simulink model "pid_adrc_duibi"  (R2023b)
settings: Solver=VariableStepAuto  StartTime=0.0  StopTime=10.0  RelTol=1e-3
values from neighbouring files (symbols this model uses):
  gama = 0.003    [startup.m]
  ke = 78.4    [startup.m]
  kf = 96.0    (= 96)    [startup.m]
  kii = 1061*R    (= 19755.82)    [startup.m]
  kiv = kpv*100    (= 7015.3125)    [startup.m]
  kp = 150    [startup.m]
  kpi = 1061*L    (= 16265.13)    [startup.m]
  kpv = 100*6*J/(kf)    (= 70.153125)    [startup.m]
  L = 15.33    [startup.m]
  R = 18.62    [startup.m]
  r = 10    [startup.m]
  tao = 0.003    [startup.m]
  U = m2^2*y^2+2*m1*m2*y^2+I1*(m1+m2)    [startup.m]
undefined symbols (not defined in the file or in its folder): sigbuilder_block
libraries: slpidlib x42, simulink x18
(part 2 of 2)

== system pid_adrc_duibi/Signal Builder1 ==
  Demux : Demux  Tag=STV Demux  Outputs=1
      settings: DisplayOption=none
  FromWs : FromWorkspace  Tag=STV FromWs  VariableName=tuvar
      SigBuilderData=|
      | common.afterFinalStr = 'Extrapolate'
      | common.sampleTime = 0
      | dataSet.timeRange = [0 10]
      | dataSet.name = 'Group 1'
      | sbobj.Groups.Name = 'Group 1'
      | sbobj.Groups.Signals.Name = 'Signal 1'
      | sbobj.Groups.Signals.XData = [0 1 2 8 9 10]
      | sbobj.Groups.Signals.YData = [0 0 1 1 1 1]
  Signal 1 : Outport  Tag=STV Outport  VectorParamsAs1DForOutWhenUnconnected=off
  wires:
  Demux/1 -> Signal 1/1
  FromWs/1 -> Demux/1

== system pid_adrc_duibi/Signal Builder2 ==
  Demux : Demux  Tag=STV Demux  Outputs=1
      settings: DisplayOption=none
  FromWs : FromWorkspace  Tag=STV FromWs  VariableName=tuvar
      SigBuilderData=|
      | common.afterFinalStr = 'Extrapolate'
      | common.sampleTime = 0
      | dataSet.timeRange = [0 10]
      | dataSet.name = 'Group 1'
      | sbobj.Groups.Name = 'Group 1'
      | sbobj.Groups.Signals.Name = 'Signal 1'
      | sbobj.Groups.Signals.XData = [0 1 2 8 9 10]
      | sbobj.Groups.Signals.YData = [0 0 1 1 1 1]
  Signal 1 : Outport  Tag=STV Outport  VectorParamsAs1DForOutWhenUnconnected=off
  wires:
  Demux/1 -> Signal 1/1
  FromWs/1 -> Demux/1

== system pid_adrc_duibi/Signal Builder3 ==
  Demux : Demux  Tag=STV Demux  Outputs=1
      settings: DisplayOption=none
  FromWs : FromWorkspace  Tag=STV FromWs  VariableName=tuvar
      SigBuilderData=|
      | common.afterFinalStr = 'Extrapolate'
      | common.sampleTime = 0
      | dataSet.timeRange = [0 10]
      | dataSet.name = 'Group 1'
      | sbobj.Groups.Name = 'Group 1'
      | sbobj.Groups.Signals.Name = 'Signal 1'
      | sbobj.Groups.Signals.XData = [0 1 2 8 9 10]
      | sbobj.Groups.Signals.YData = [0 0 1 1 1 1]
  Signal 1 : Outport  Tag=STV Outport  VectorParamsAs1DForOutWhenUnconnected=off
  wires:
  Demux/1 -> Signal 1/1
  FromWs/1 -> Demux/1

== system pid_adrc_duibi/Signal Builder4 ==
  Demux : Demux  Tag=STV Demux  Outputs=1
      settings: DisplayOption=none
  FromWs : FromWorkspace  Tag=STV FromWs  VariableName=tuvar
      SigBuilderData=|
      | common.afterFinalStr = 'Extrapolate'
      | common.sampleTime = 0
      | dataSet.timeRange = [0 10]
      | dataSet.name = 'Group 1'
      | sbobj.Groups.Name = 'Group 1'
      | sbobj.Groups.Signals.Name = 'Signal 1'
      | sbobj.Groups.Signals.XData = [0 1 2 8 9 10]
      | sbobj.Groups.Signals.YData = [0 0 1 1 1 1]
  Signal 1 : Outport  Tag=STV Outport  VectorParamsAs1DForOutWhenUnconnected=off
  wires:
  Demux/1 -> Signal 1/1
  FromWs/1 -> Demux/1

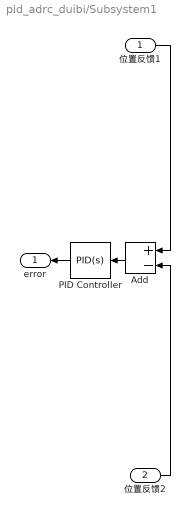
== system pid_adrc_duibi/Subsystem1 ==
  位置反馈1 : Inport
  位置反馈2 : Inport  Port=2
  Add : Sum  Inputs=+-
  PID Controller : simulink/Continuous/PID Controller  Controller=PID  TimeDomain=Continuous-time  SampleTime=-1  IntegratorMethod=Forward Euler  FilterMethod=Forward Euler  Form=Parallel  UseFilter=on  ControllerParametersSource=internal  P=e_kp  I=e_ki  D=e_kd  N=100  InitialConditionSource=internal  InitialConditionForIntegrator=0  InitialConditionForFilter=0  ExternalReset=none  LimitOutput=off  UpperSaturationLimit=inf  LowerSaturationLimit=-inf  LinearizeAsGain=on  AntiWindupMode=none  Kb=1  TrackingMode=off  Kt=1  PParamMin=[]  PParamMax=[]  IParamMin=[]  IParamMax=[]  DParamMin=[]  DParamMax=[]  NParamMin=[]  NParamMax=[]  KbParamMin=[]  KbParamMax=[]  KtParamMin=[]  KtParamMax=[]  POutMin=[]  POutMax=[]  IOutMin=[]  IOutMax=[]  DOutMin=[]  DOutMax=[]  NOutMin=[]  NOutMax=[]  KbOutMin=[]  KbOutMax=[]  KtOutMin=[]  KtOutMax=[]  IntegratorOutMin=[]  IntegratorOutMax=[]  FilterOutMin=[]  FilterOutMax=[]  SumOutMin=[]  SumOutMax=[]  SumI1OutMin=[]  SumI1OutMax=[]  SumI2OutMin=[]  SumI2OutMax=[]  SumI3OutMin=[]  SumI3OutMax=[]  SumDOutMin=[]  SumDOutMax=[]  SaturationOutMin=[]  SaturationOutMax=[]  IntegratorContinuousStateAttributes=''  IntegratorStateMustResolveToSignalObject=off  IntegratorRTWStateStorageClass=Auto  FilterContinuousStateAttributes=''  FilterStateMustResolveToSignalObject=off  FilterRTWStateStorageClass=Auto  DifferentiatorICPrevScaledInput=0  DifferentiatorOutMin=[]  DifferentiatorOutMax=[]  FilterDiffOutCoefMin=[]  FilterDiffOutCoefMax=[]  SumDenOutMin=[]  SumDenOutMax=[]  SumNumOutMin=[]  SumNumOutMax=[]  ReciprocalOutMin=[]  ReciprocalOutMax=[]  DivideOutMin=[]  DivideOutMax=[]  TunerSelectOption=Transfer Function Based (PID Tuner App)
  error : Outport  VectorParamsAs1DForOutWhenUnconnected=off
  wires:
  位置反馈2/1 -> Add/2
  Add/1 -> PID Controller/1
  PID Controller/1 -> error/1
  位置反馈1/1 -> Add/1

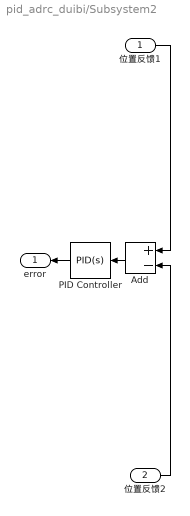
== system pid_adrc_duibi/Subsystem2 ==
  位置反馈1 : Inport
  位置反馈2 : Inport  Port=2
  Add : Sum  Inputs=+-
  PID Controller : slpidlib/PID Controller  Controller=PID  Form=Parallel  TimeDomain=Continuous-time  UseExternalTs=off  SampleTime=-1  IntegratorMethod=Forward Euler  FilterMethod=Forward Euler  ControllerParametersSource=internal  P=e_kp  I=e_ki  UseKiTs=off  D=e_kd  N=100  UseFilter=on  TunerSelectOption=Transfer Function Based (PID Tuner App)  InitialConditionSource=internal  InitialConditionForIntegrator=0  InitialConditionForFilter=0  DifferentiatorICPrevScaledInput=0  ExternalReset=none  TrackingMode=off  Kt=1  LimitOutput=off  SatLimitsSource=internal  UpperSaturationLimit=inf  LowerSaturationLimit=-inf  LinearizeAsGain=on  AntiWindupMode=none  Kb=1  LimitIntegrator=off  UpperIntegratorSaturationLimit=inf  LowerIntegratorSaturationLimit=-inf  POutMin=[]  POutMax=[]  IOutMin=[]  IOutMax=[]  DOutMin=[]  DOutMax=[]  NOutMin=[]  NOutMax=[]  SumOutMin=[]  SumOutMax=[]  SaturationOutMin=[]  SaturationOutMax=[]  PParamMin=[]  PParamMax=[]  IParamMin=[]  IParamMax=[]  DParamMin=[]  DParamMax=[]  NParamMin=[]  NParamMax=[]  KbParamMin=[]  KbParamMax=[]  KtParamMin=[]  KtParamMax=[]  KbOutMin=[]  KbOutMax=[]  KtOutMin=[]  KtOutMax=[]  IntegratorOutMin=[]  IntegratorOutMax=[]  FilterOutMin=[]  FilterOutMax=[]  SumI1OutMin=[]  SumI1OutMax=[]  SumI2OutMin=[]  SumI2OutMax=[]  SumI3OutMin=[]  SumI3OutMax=[]  SumI4OutMin=[]  SumI4OutMax=[]  SumDOutMin=[]  SumDOutMax=[]  DifferentiatorOutMin=[]  DifferentiatorOutMax=[]  FilterDiffOutCoefMin=[]  FilterDiffOutCoefMax=[]  ReciprocalOutMin=[]  ReciprocalOutMax=[]  SumDenOutMin=[]  SumDenOutMax=[]  SumNumOutMin=[]  SumNumOutMax=[]  DivideOutMin=[]  DivideOutMax=[]  UdiffTsProdOutMin=[]  UdiffTsProdOutMax=[]  NTsProdOutMin=[]  NTsProdOutMax=[]  UintegralTsProdOutMin=[]  UintegralTsProdOutMax=[]  UngainTsProdOutMin=[]  UngainTsProdOutMax=[]  ClampingZeroOutDataTypeStr=Inherit: Inherit via back propagation  ClampingZeroOutMin=[]  ClampingZeroOutMax=[]  FilterDenConstantOutDataTypeStr=Inherit: Inherit via back propagation  FilterDenConstantOutMin=[]  FilterDenConstantOutMax=[]  PCopyOutDataTypeStr=Inherit: Inherit via back propagation  PCopyOutMin=[]  PCopyOutMax=[]  NCopyOutDataTypeStr=Inherit: Inherit via back propagation  NCopyOutMin=[]  NCopyOutMax=[]  IntegratorContinuousStateAttributes=''  IntegratorStateMustResolveToSignalObject=off  IntegratorRTWStateStorageClass=Auto  FilterContinuousStateAttributes=''  FilterStateMustResolveToSignalObject=off  FilterRTWStateStorageClass=Auto  ParallelPVariant=InternalParameters  IdealPVariant=Disabled  IVariant=InternalParameters  DVariant=InternalParameters  IntegratorVariant=Continuous  SatVariant=Disabled  AWVariant=Passthrough  PCopyVariant=Disabled  TRVariant=Disabled  FdbkBlocksVariant=Forward  IdealPFdbkVariant=Disabled  SatFdbkVariant=Disabled  DerivativeFilterVariant=ContFilter  NVariant=InternalParameters  NCopyVariant=Disabled  FilterICVariant=InternalICsFilter  IntegratorICVariant=InternalICs  ExternalResetVariant=Disabled  TRSumVariant=Passthrough  SumFdbkVariant=Disabled  SumVariant=Sum_PID  TsampFilterVariant=InternalTs  TsampNgainVariant=Passthrough  TsampIntegralVariant=Disabled_SignalSpec  ExternalSaturationOutDataTypeStr=Inherit: Same as second input
  error : Outport  VectorParamsAs1DForOutWhenUnconnected=off
  wires:
  位置反馈2/1 -> Add/2
  Add/1 -> PID Controller/1
  PID Controller/1 -> error/1
  位置反馈1/1 -> Add/1

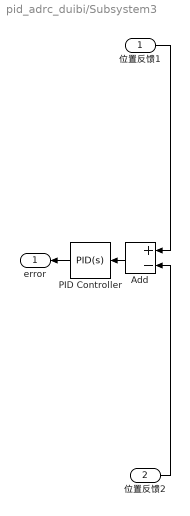
== system pid_adrc_duibi/Subsystem3 ==
  位置反馈1 : Inport
  位置反馈2 : Inport  Port=2
  Add : Sum  Inputs=+-
  PID Controller : slpidlib/PID Controller  Controller=PID  Form=Parallel  TimeDomain=Continuous-time  UseExternalTs=off  SampleTime=-1  IntegratorMethod=Forward Euler  FilterMethod=Forward Euler  ControllerParametersSource=internal  P=e_kp  I=e_ki  UseKiTs=off  D=e_kd  N=100  UseFilter=on  TunerSelectOption=Transfer Function Based (PID Tuner App)  InitialConditionSource=internal  InitialConditionForIntegrator=0  InitialConditionForFilter=0  DifferentiatorICPrevScaledInput=0  ExternalReset=none  TrackingMode=off  Kt=1  LimitOutput=off  SatLimitsSource=internal  UpperSaturationLimit=inf  LowerSaturationLimit=-inf  LinearizeAsGain=on  AntiWindupMode=none  Kb=1  LimitIntegrator=off  UpperIntegratorSaturationLimit=inf  LowerIntegratorSaturationLimit=-inf  POutMin=[]  POutMax=[]  IOutMin=[]  IOutMax=[]  DOutMin=[]  DOutMax=[]  NOutMin=[]  NOutMax=[]  SumOutMin=[]  SumOutMax=[]  SaturationOutMin=[]  SaturationOutMax=[]  PParamMin=[]  PParamMax=[]  IParamMin=[]  IParamMax=[]  DParamMin=[]  DParamMax=[]  NParamMin=[]  NParamMax=[]  KbParamMin=[]  KbParamMax=[]  KtParamMin=[]  KtParamMax=[]  KbOutMin=[]  KbOutMax=[]  KtOutMin=[]  KtOutMax=[]  IntegratorOutMin=[]  IntegratorOutMax=[]  FilterOutMin=[]  FilterOutMax=[]  SumI1OutMin=[]  SumI1OutMax=[]  SumI2OutMin=[]  SumI2OutMax=[]  SumI3OutMin=[]  SumI3OutMax=[]  SumI4OutMin=[]  SumI4OutMax=[]  SumDOutMin=[]  SumDOutMax=[]  DifferentiatorOutMin=[]  DifferentiatorOutMax=[]  FilterDiffOutCoefMin=[]  FilterDiffOutCoefMax=[]  ReciprocalOutMin=[]  ReciprocalOutMax=[]  SumDenOutMin=[]  SumDenOutMax=[]  SumNumOutMin=[]  SumNumOutMax=[]  DivideOutMin=[]  DivideOutMax=[]  UdiffTsProdOutMin=[]  UdiffTsProdOutMax=[]  NTsProdOutMin=[]  NTsProdOutMax=[]  UintegralTsProdOutMin=[]  UintegralTsProdOutMax=[]  UngainTsProdOutMin=[]  UngainTsProdOutMax=[]  ClampingZeroOutDataTypeStr=Inherit: Inherit via back propagation  ClampingZeroOutMin=[]  ClampingZeroOutMax=[]  FilterDenConstantOutDataTypeStr=Inherit: Inherit via back propagation  FilterDenConstantOutMin=[]  FilterDenConstantOutMax=[]  PCopyOutDataTypeStr=Inherit: Inherit via back propagation  PCopyOutMin=[]  PCopyOutMax=[]  NCopyOutDataTypeStr=Inherit: Inherit via back propagation  NCopyOutMin=[]  NCopyOutMax=[]  IntegratorContinuousStateAttributes=''  IntegratorStateMustResolveToSignalObject=off  IntegratorRTWStateStorageClass=Auto  FilterContinuousStateAttributes=''  FilterStateMustResolveToSignalObject=off  FilterRTWStateStorageClass=Auto  ParallelPVariant=InternalParameters  IdealPVariant=Disabled  IVariant=InternalParameters  DVariant=InternalParameters  IntegratorVariant=Continuous  SatVariant=Disabled  AWVariant=Passthrough  PCopyVariant=Disabled  TRVariant=Disabled  FdbkBlocksVariant=Forward  IdealPFdbkVariant=Disabled  SatFdbkVariant=Disabled  DerivativeFilterVariant=ContFilter  NVariant=InternalParameters  NCopyVariant=Disabled  FilterICVariant=InternalICsFilter  IntegratorICVariant=InternalICs  ExternalResetVariant=Disabled  TRSumVariant=Passthrough  SumFdbkVariant=Disabled  SumVariant=Sum_PID  TsampFilterVariant=InternalTs  TsampNgainVariant=Passthrough  TsampIntegralVariant=Disabled_SignalSpec  ExternalSaturationOutDataTypeStr=Inherit: Same as second input
  error : Outport  VectorParamsAs1DForOutWhenUnconnected=off
  wires:
  位置反馈2/1 -> Add/2
  Add/1 -> PID Controller/1
  PID Controller/1 -> error/1
  位置反馈1/1 -> Add/1

== system pid_adrc_duibi/Subsystem4 ==
  位置反馈1 : Inport
  位置反馈2 : Inport  Port=2
  Add : Sum  Inputs=+-
  PID Controller : simulink/Continuous/PID Controller  Controller=PID  TimeDomain=Continuous-time  SampleTime=-1  IntegratorMethod=Forward Euler  FilterMethod=Forward Euler  Form=Parallel  UseFilter=on  ControllerParametersSource=internal  P=e_kp  I=e_ki  D=e_kd  N=100  InitialConditionSource=internal  InitialConditionForIntegrator=0  InitialConditionForFilter=0  ExternalReset=none  LimitOutput=off  UpperSaturationLimit=inf  LowerSaturationLimit=-inf  LinearizeAsGain=on  AntiWindupMode=none  Kb=1  TrackingMode=off  Kt=1  PParamMin=[]  PParamMax=[]  IParamMin=[]  IParamMax=[]  DParamMin=[]  DParamMax=[]  NParamMin=[]  NParamMax=[]  KbParamMin=[]  KbParamMax=[]  KtParamMin=[]  KtParamMax=[]  POutMin=[]  POutMax=[]  IOutMin=[]  IOutMax=[]  DOutMin=[]  DOutMax=[]  NOutMin=[]  NOutMax=[]  KbOutMin=[]  KbOutMax=[]  KtOutMin=[]  KtOutMax=[]  IntegratorOutMin=[]  IntegratorOutMax=[]  FilterOutMin=[]  FilterOutMax=[]  SumOutMin=[]  SumOutMax=[]  SumI1OutMin=[]  SumI1OutMax=[]  SumI2OutMin=[]  SumI2OutMax=[]  SumI3OutMin=[]  SumI3OutMax=[]  SumDOutMin=[]  SumDOutMax=[]  SaturationOutMin=[]  SaturationOutMax=[]  IntegratorContinuousStateAttributes=''  IntegratorStateMustResolveToSignalObject=off  IntegratorRTWStateStorageClass=Auto  FilterContinuousStateAttributes=''  FilterStateMustResolveToSignalObject=off  FilterRTWStateStorageClass=Auto  DifferentiatorICPrevScaledInput=0  DifferentiatorOutMin=[]  DifferentiatorOutMax=[]  FilterDiffOutCoefMin=[]  FilterDiffOutCoefMax=[]  SumDenOutMin=[]  SumDenOutMax=[]  SumNumOutMin=[]  SumNumOutMax=[]  ReciprocalOutMin=[]  ReciprocalOutMax=[]  DivideOutMin=[]  DivideOutMax=[]  TunerSelectOption=Transfer Function Based (PID Tuner App)
  error : Outport  VectorParamsAs1DForOutWhenUnconnected=off
  wires:
  位置反馈2/1 -> Add/2
  Add/1 -> PID Controller/1
  PID Controller/1 -> error/1
  位置反馈1/1 -> Add/1

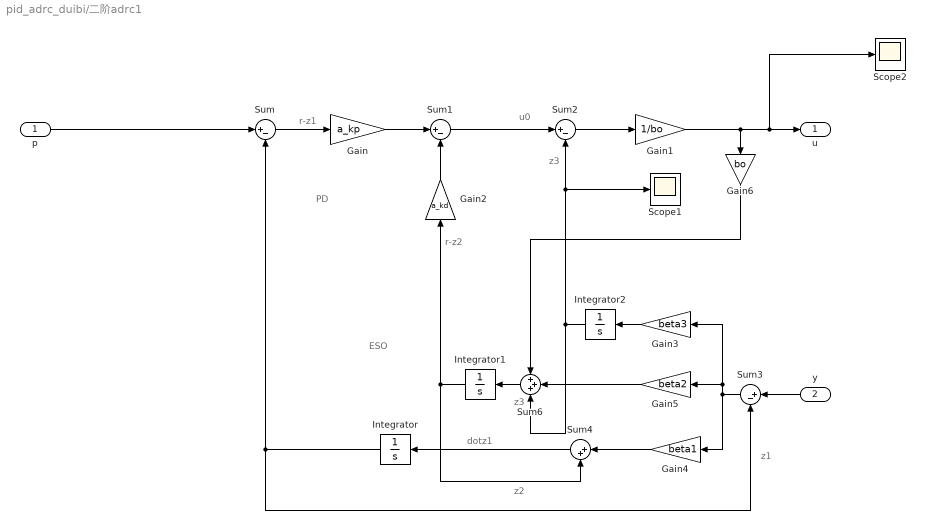
== system pid_adrc_duibi/二阶adrc1 ==
  note: ESO
  note: PD
  note: z3
  note: dotz1
  note: z2
  note: z1
  note: z3
  note: u0
  note: r-z2
  note: r-z1
  p : Inport
  y : Inport  Port=2
  Gain : Gain  Gain=a_kp
  Gain1 : Gain  Gain=1/bo
  Gain2 : Gain  Gain=a_kd
  Gain3 : Gain  Gain=beta3
  Gain4 : Gain  Gain=beta1
  Gain5 : Gain  Gain=beta2
  Gain6 : Gain  Gain=bo
  Integrator : Integrator
  Integrator1 : Integrator
  Integrator2 : Integrator
  Scope1 : Scope
  Scope2 : Scope
  Sum{,1..3} (4 alike) : Sum  Inputs=|+-
  Sum4 : Sum  Inputs=|++
  Sum6 : Sum  Inputs=+++
  u : Outport  VectorParamsAs1DForOutWhenUnconnected=off
  wires:
  p/1 -> Sum/1
  Sum/1 -> Gain/1
  Gain/1 -> Sum1/1
  Gain2/1 -> Sum1/2
  Sum2/1 -> Gain1/1
  Gain1/1 -> Gain6/1, Scope2/1, u/1
  Integrator/1 -> Sum/2, Sum3/2
  y/1 -> Sum3/1
  Sum3/1 -> Gain4/1, Gain3/1, Gain5/1
  Gain4/1 -> Sum4/1
  Sum4/1 -> Integrator/1
  Gain5/1 -> Sum6/2
  Gain6/1 -> Sum6/1
  Integrator2/1 -> Sum6/3, Sum2/2, Scope1/1
  Sum6/1 -> Integrator1/1
  Gain3/1 -> Integrator2/1
  Integrator1/1 -> Gain2/1, Sum4/2
  Sum1/1 -> Sum2/1

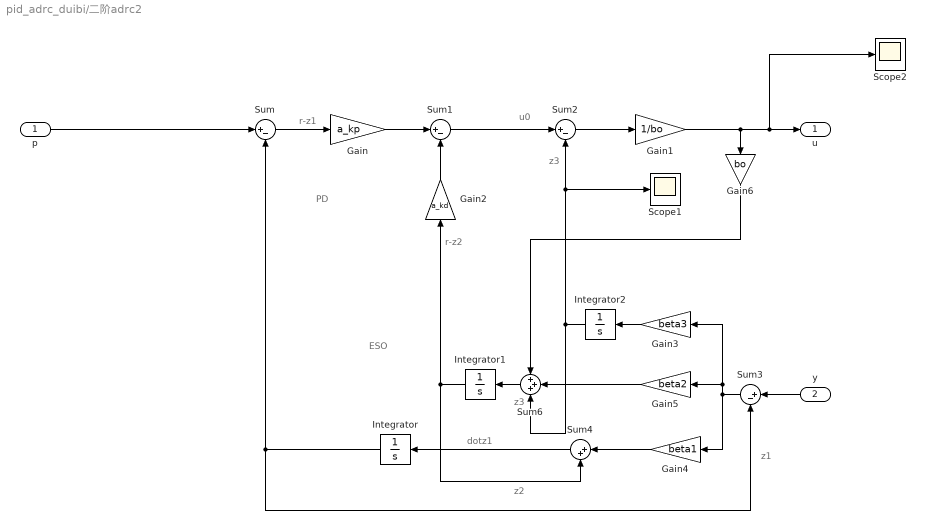
== system pid_adrc_duibi/二阶adrc2 ==
  note: ESO
  note: PD
  note: z3
  note: dotz1
  note: z2
  note: z1
  note: z3
  note: u0
  note: r-z2
  note: r-z1
  p : Inport
  y : Inport  Port=2
  Gain : Gain  Gain=a_kp
  Gain1 : Gain  Gain=1/bo
  Gain2 : Gain  Gain=a_kd
  Gain3 : Gain  Gain=beta3
  Gain4 : Gain  Gain=beta1
  Gain5 : Gain  Gain=beta2
  Gain6 : Gain  Gain=bo
  Integrator : Integrator
  Integrator1 : Integrator
  Integrator2 : Integrator
  Scope1 : Scope
  Scope2 : Scope
  Sum{,1..3} (4 alike) : Sum  Inputs=|+-
  Sum4 : Sum  Inputs=|++
  Sum6 : Sum  Inputs=+++
  u : Outport  VectorParamsAs1DForOutWhenUnconnected=off
  wires:
  p/1 -> Sum/1
  Sum/1 -> Gain/1
  Gain/1 -> Sum1/1
  Gain2/1 -> Sum1/2
  Sum2/1 -> Gain1/1
  Gain1/1 -> Gain6/1, Scope2/1, u/1
  Integrator/1 -> Sum/2, Sum3/2
  y/1 -> Sum3/1
  Sum3/1 -> Gain4/1, Gain3/1, Gain5/1
  Gain4/1 -> Sum4/1
  Sum4/1 -> Integrator/1
  Gain5/1 -> Sum6/2
  Gain6/1 -> Sum6/1
  Integrator2/1 -> Sum6/3, Sum2/2, Scope1/1
  Sum6/1 -> Integrator1/1
  Gain3/1 -> Integrator2/1
  Sum1/1 -> Sum2/1
  Integrator1/1 -> Gain2/1, Sum4/2

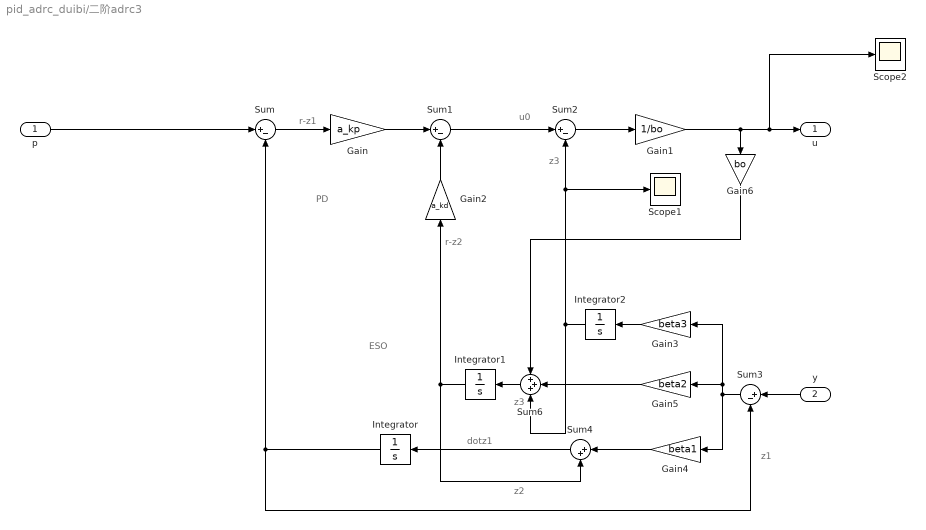
== system pid_adrc_duibi/二阶adrc3 ==
  note: ESO
  note: PD
  note: z3
  note: dotz1
  note: z2
  note: z1
  note: z3
  note: u0
  note: r-z2
  note: r-z1
  p : Inport
  y : Inport  Port=2
  Gain : Gain  Gain=a_kp
  Gain1 : Gain  Gain=1/bo
  Gain2 : Gain  Gain=a_kd
  Gain3 : Gain  Gain=beta3
  Gain4 : Gain  Gain=beta1
  Gain5 : Gain  Gain=beta2
  Gain6 : Gain  Gain=bo
  Integrator : Integrator
  Integrator1 : Integrator
  Integrator2 : Integrator
  Scope1 : Scope
  Scope2 : Scope
  Sum{,1..3} (4 alike) : Sum  Inputs=|+-
  Sum4 : Sum  Inputs=|++
  Sum6 : Sum  Inputs=+++
  u : Outport  VectorParamsAs1DForOutWhenUnconnected=off
  wires:
  p/1 -> Sum/1
  Sum/1 -> Gain/1
  Gain/1 -> Sum1/1
  Gain2/1 -> Sum1/2
  Sum2/1 -> Gain1/1
  Gain1/1 -> Gain6/1, Scope2/1, u/1
  Integrator/1 -> Sum/2, Sum3/2
  y/1 -> Sum3/1
  Sum3/1 -> Gain4/1, Gain3/1, Gain5/1
  Gain4/1 -> Sum4/1
  Sum4/1 -> Integrator/1
  Gain5/1 -> Sum6/2
  Gain6/1 -> Sum6/1
  Integrator2/1 -> Sum6/3, Sum2/2, Scope1/1
  Sum6/1 -> Integrator1/1
  Gain3/1 -> Integrator2/1
  Integrator1/1 -> Gain2/1, Sum4/2
  Sum1/1 -> Sum2/1

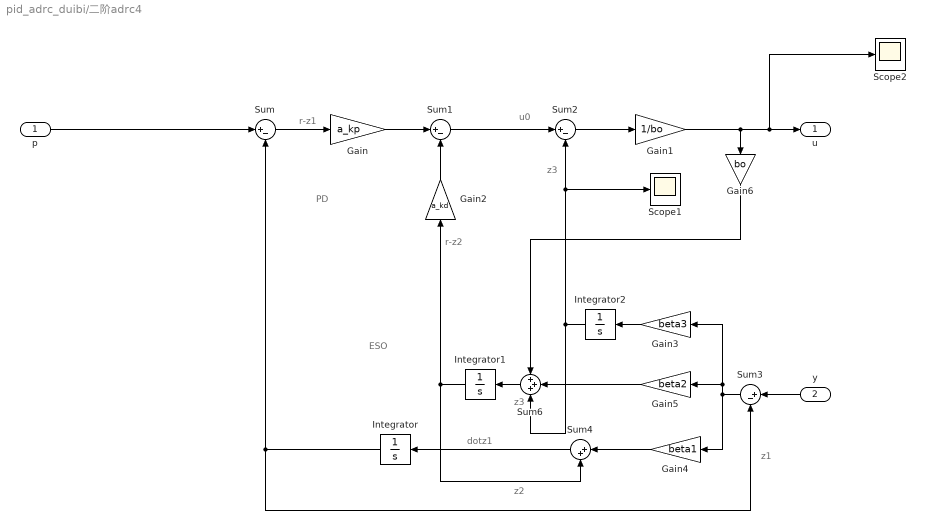
== system pid_adrc_duibi/二阶adrc4 ==
  note: ESO
  note: PD
  note: z3
  note: dotz1
  note: z2
  note: z1
  note: z3
  note: u0
  note: r-z2
  note: r-z1
  p : Inport
  y : Inport  Port=2
  Gain : Gain  Gain=a_kp
  Gain1 : Gain  Gain=1/bo
  Gain2 : Gain  Gain=a_kd
  Gain3 : Gain  Gain=beta3
  Gain4 : Gain  Gain=beta1
  Gain5 : Gain  Gain=beta2
  Gain6 : Gain  Gain=bo
  Integrator : Integrator
  Integrator1 : Integrator
  Integrator2 : Integrator
  Scope1 : Scope
  Scope2 : Scope
  Sum{,1..3} (4 alike) : Sum  Inputs=|+-
  Sum4 : Sum  Inputs=|++
  Sum6 : Sum  Inputs=+++
  u : Outport  VectorParamsAs1DForOutWhenUnconnected=off
  wires:
  Sum/1 -> Gain/1
  Gain/1 -> Sum1/1
  Gain2/1 -> Sum1/2
  Sum2/1 -> Gain1/1
  Gain1/1 -> Gain6/1, Scope2/1, u/1
  Integrator/1 -> Sum/2, Sum3/2
  y/1 -> Sum3/1
  Sum3/1 -> Gain4/1, Gain3/1, Gain5/1
  Gain4/1 -> Sum4/1
  Sum4/1 -> Integrator/1
  Gain5/1 -> Sum6/2
  Gain6/1 -> Sum6/1
  Integrator2/1 -> Sum6/3, Sum2/2, Scope1/1
  Sum6/1 -> Integrator1/1
  Gain3/1 -> Integrator2/1
  Integrator1/1 -> Gain2/1, Sum4/2
  p/1 -> Sum/1
  Sum1/1 -> Sum2/1

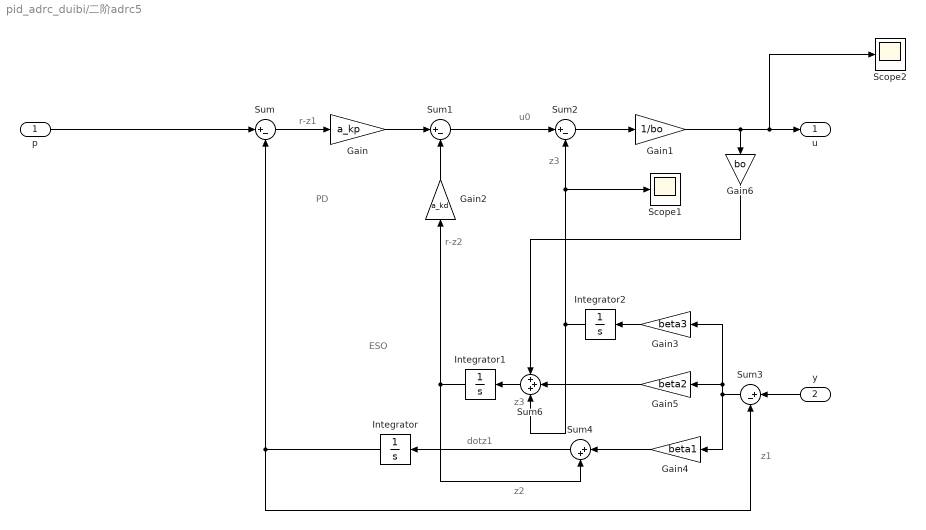
== system pid_adrc_duibi/二阶adrc5 ==
  note: ESO
  note: PD
  note: z3
  note: dotz1
  note: z2
  note: z1
  note: z3
  note: u0
  note: r-z2
  note: r-z1
  p : Inport
  y : Inport  Port=2
  Gain : Gain  Gain=a_kp
  Gain1 : Gain  Gain=1/bo
  Gain2 : Gain  Gain=a_kd
  Gain3 : Gain  Gain=beta3
  Gain4 : Gain  Gain=beta1
  Gain5 : Gain  Gain=beta2
  Gain6 : Gain  Gain=bo
  Integrator : Integrator
  Integrator1 : Integrator
  Integrator2 : Integrator
  Scope1 : Scope
  Scope2 : Scope
  Sum{,1..3} (4 alike) : Sum  Inputs=|+-
  Sum4 : Sum  Inputs=|++
  Sum6 : Sum  Inputs=+++
  u : Outport  VectorParamsAs1DForOutWhenUnconnected=off
  wires:
  p/1 -> Sum/1
  Sum/1 -> Gain/1
  Gain/1 -> Sum1/1
  Gain2/1 -> Sum1/2
  Sum2/1 -> Gain1/1
  Gain1/1 -> Gain6/1, Scope2/1, u/1
  Integrator/1 -> Sum/2, Sum3/2
  y/1 -> Sum3/1
  Sum3/1 -> Gain4/1, Gain3/1, Gain5/1
  Gain4/1 -> Sum4/1
  Sum4/1 -> Integrator/1
  Gain5/1 -> Sum6/2
  Gain6/1 -> Sum6/1
  Integrator2/1 -> Sum6/3, Sum2/2, Scope1/1
  Sum6/1 -> Integrator1/1
  Gain3/1 -> Integrator2/1
  Sum1/1 -> Sum2/1
  Integrator1/1 -> Gain2/1, Sum4/2

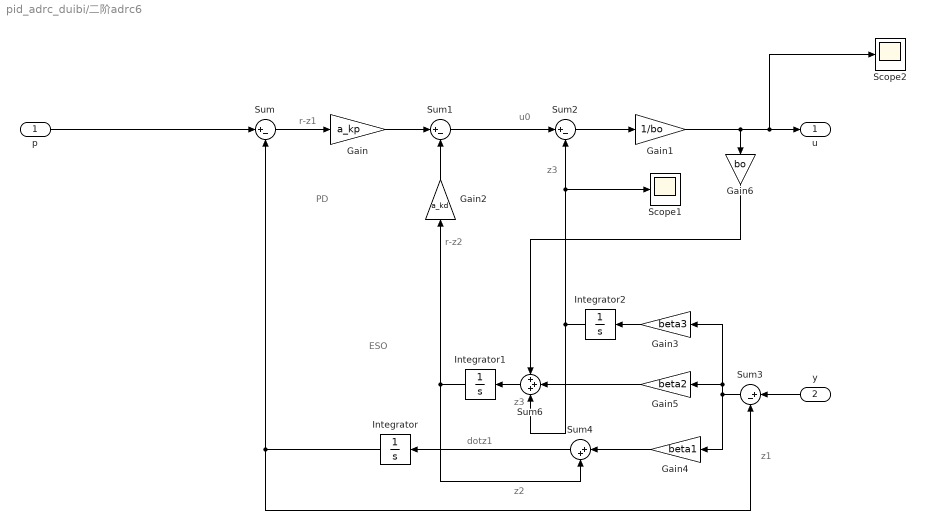
== system pid_adrc_duibi/二阶adrc6 ==
  note: ESO
  note: PD
  note: z3
  note: dotz1
  note: z2
  note: z1
  note: z3
  note: u0
  note: r-z2
  note: r-z1
  p : Inport
  y : Inport  Port=2
  Gain : Gain  Gain=a_kp
  Gain1 : Gain  Gain=1/bo
  Gain2 : Gain  Gain=a_kd
  Gain3 : Gain  Gain=beta3
  Gain4 : Gain  Gain=beta1
  Gain5 : Gain  Gain=beta2
  Gain6 : Gain  Gain=bo
  Integrator : Integrator
  Integrator1 : Integrator
  Integrator2 : Integrator
  Scope1 : Scope
  Scope2 : Scope
  Sum{,1..3} (4 alike) : Sum  Inputs=|+-
  Sum4 : Sum  Inputs=|++
  Sum6 : Sum  Inputs=+++
  u : Outport  VectorParamsAs1DForOutWhenUnconnected=off
  wires:
  Sum/1 -> Gain/1
  Gain/1 -> Sum1/1
  Gain2/1 -> Sum1/2
  Sum2/1 -> Gain1/1
  Gain1/1 -> Gain6/1, Scope2/1, u/1
  Integrator/1 -> Sum/2, Sum3/2
  y/1 -> Sum3/1
  Sum3/1 -> Gain4/1, Gain3/1, Gain5/1
  Gain4/1 -> Sum4/1
  Sum4/1 -> Integrator/1
  Gain5/1 -> Sum6/2
  Gain6/1 -> Sum6/1
  Integrator2/1 -> Sum6/3, Sum2/2, Scope1/1
  Sum6/1 -> Integrator1/1
  Gain3/1 -> Integrator2/1
  Integrator1/1 -> Gain2/1, Sum4/2
  p/1 -> Sum/1
  Sum1/1 -> Sum2/1

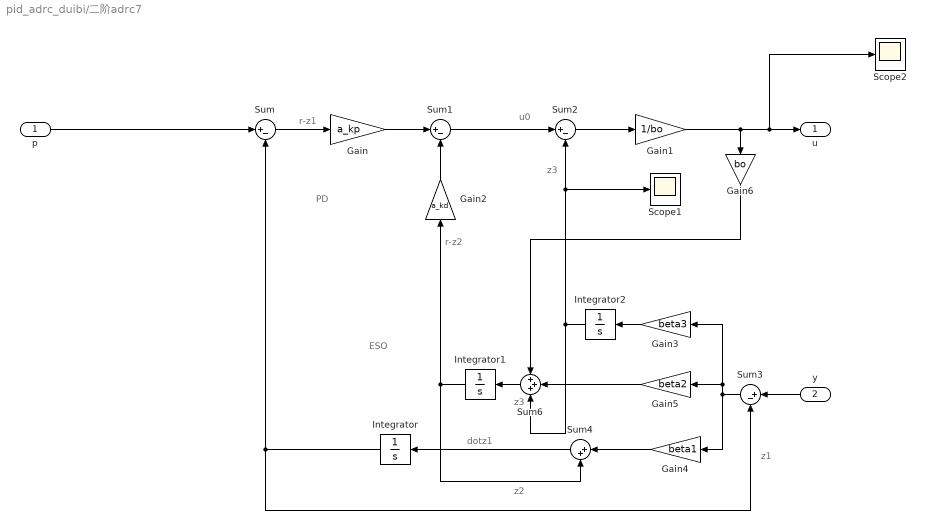
== system pid_adrc_duibi/二阶adrc7 ==
  note: ESO
  note: PD
  note: z3
  note: dotz1
  note: z2
  note: z1
  note: z3
  note: u0
  note: r-z2
  note: r-z1
  p : Inport
  y : Inport  Port=2
  Gain : Gain  Gain=a_kp
  Gain1 : Gain  Gain=1/bo
  Gain2 : Gain  Gain=a_kd
  Gain3 : Gain  Gain=beta3
  Gain4 : Gain  Gain=beta1
  Gain5 : Gain  Gain=beta2
  Gain6 : Gain  Gain=bo
  Integrator : Integrator
  Integrator1 : Integrator
  Integrator2 : Integrator
  Scope1 : Scope
  Scope2 : Scope
  Sum{,1..3} (4 alike) : Sum  Inputs=|+-
  Sum4 : Sum  Inputs=|++
  Sum6 : Sum  Inputs=+++
  u : Outport  VectorParamsAs1DForOutWhenUnconnected=off
  wires:
  Sum/1 -> Gain/1
  Gain/1 -> Sum1/1
  Gain2/1 -> Sum1/2
  Sum2/1 -> Gain1/1
  Gain1/1 -> Gain6/1, Scope2/1, u/1
  Integrator/1 -> Sum/2, Sum3/2
  y/1 -> Sum3/1
  Sum3/1 -> Gain4/1, Gain3/1, Gain5/1
  Gain4/1 -> Sum4/1
  Sum4/1 -> Integrator/1
  Gain5/1 -> Sum6/2
  Gain6/1 -> Sum6/1
  Integrator2/1 -> Sum6/3, Sum2/2, Scope1/1
  Sum6/1 -> Integrator1/1
  Gain3/1 -> Integrator2/1
  Integrator1/1 -> Gain2/1, Sum4/2
  p/1 -> Sum/1
  Sum1/1 -> Sum2/1

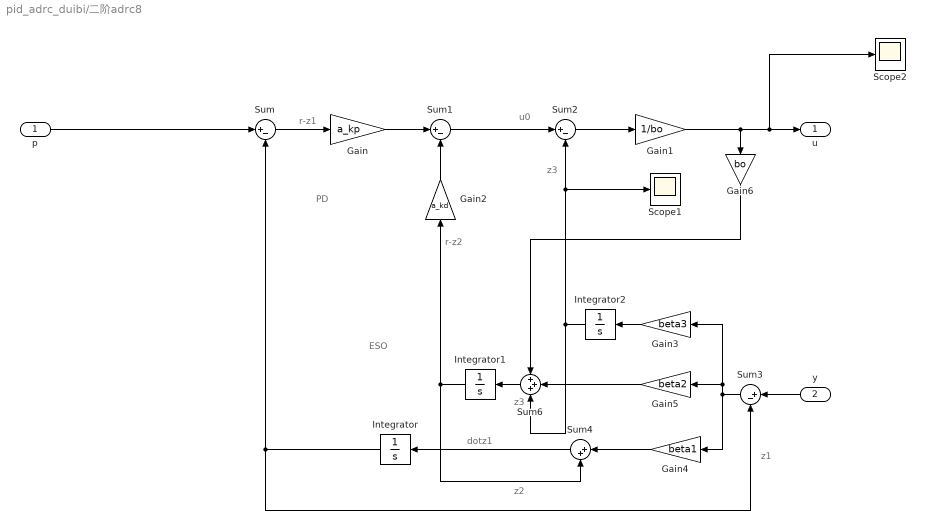
== system pid_adrc_duibi/二阶adrc8 ==
  note: ESO
  note: PD
  note: z3
  note: dotz1
  note: z2
  note: z1
  note: z3
  note: u0
  note: r-z2
  note: r-z1
  p : Inport
  y : Inport  Port=2
  Gain : Gain  Gain=a_kp
  Gain1 : Gain  Gain=1/bo
  Gain2 : Gain  Gain=a_kd
  Gain3 : Gain  Gain=beta3
  Gain4 : Gain  Gain=beta1
  Gain5 : Gain  Gain=beta2
  Gain6 : Gain  Gain=bo
  Integrator : Integrator
  Integrator1 : Integrator
  Integrator2 : Integrator
  Scope1 : Scope
  Scope2 : Scope
  Sum{,1..3} (4 alike) : Sum  Inputs=|+-
  Sum4 : Sum  Inputs=|++
  Sum6 : Sum  Inputs=+++
  u : Outport  VectorParamsAs1DForOutWhenUnconnected=off
  wires:
  Sum/1 -> Gain/1
  Gain/1 -> Sum1/1
  Gain2/1 -> Sum1/2
  Sum2/1 -> Gain1/1
  Gain1/1 -> Gain6/1, Scope2/1, u/1
  Integrator/1 -> Sum/2, Sum3/2
  y/1 -> Sum3/1
  Sum3/1 -> Gain4/1, Gain3/1, Gain5/1
  Gain4/1 -> Sum4/1
  Sum4/1 -> Integrator/1
  Gain5/1 -> Sum6/2
  Gain6/1 -> Sum6/1
  Integrator2/1 -> Sum6/3, Sum2/2, Scope1/1
  Sum6/1 -> Integrator1/1
  Gain3/1 -> Integrator2/1
  Integrator1/1 -> Gain2/1, Sum4/2
  p/1 -> Sum/1
  Sum1/1 -> Sum2/1

== system pid_adrc_duibi/同 ==
  Step20 : Step  Time=3  After=r  SampleTime=0
  Step24 : Step  Time=4  After=-r  SampleTime=0
  Sum96 : Sum  Inputs=++|
  Out1 : Outport
  wires:
  Step24/1 -> Sum96/2
  Step20/1 -> Sum96/1
  Sum96/1 -> Out1/1

== system pid_adrc_duibi/同1 ==
  Step20 : Step  Time=3  After=r  SampleTime=0
  Step24 : Step  Time=4  After=-r  SampleTime=0
  Sum96 : Sum  Inputs=++|
  Out1 : Outport
  wires:
  Step24/1 -> Sum96/2
  Step20/1 -> Sum96/1
  Sum96/1 -> Out1/1

== system pid_adrc_duibi/同2 ==
  Step20 : Step  Time=3  After=r  SampleTime=0
  Step24 : Step  Time=4  After=-r  SampleTime=0
  Sum96 : Sum  Inputs=++|
  Out1 : Outport
  wires:
  Step24/1 -> Sum96/2
  Step20/1 -> Sum96/1
  Sum96/1 -> Out1/1

== system pid_adrc_duibi/同3 ==
  Step20 : Step  Time=3  After=r  SampleTime=0
  Step24 : Step  Time=4  After=-r  SampleTime=0
  Sum96 : Sum  Inputs=++|
  Out1 : Outport
  wires:
  Step24/1 -> Sum96/2
  Step20/1 -> Sum96/1
  Sum96/1 -> Out1/1

== system pid_adrc_duibi/同4 ==
  Step20 : Step  Time=3  After=r  SampleTime=0
  Step24 : Step  Time=4  After=-r  SampleTime=0
  Sum96 : Sum  Inputs=++|
  Out1 : Outport
  wires:
  Step24/1 -> Sum96/2
  Step20/1 -> Sum96/1
  Sum96/1 -> Out1/1

== system pid_adrc_duibi/同5 ==
  Step20 : Step  Time=3  After=r  SampleTime=0
  Step24 : Step  Time=4  After=-r  SampleTime=0
  Sum96 : Sum  Inputs=++|
  Out1 : Outport
  wires:
  Step24/1 -> Sum96/2
  Step20/1 -> Sum96/1
  Sum96/1 -> Out1/1

== system pid_adrc_duibi/同6 ==
  Step20 : Step  Time=3  After=r  SampleTime=0
  Step24 : Step  Time=4  After=-r  SampleTime=0
  Sum96 : Sum  Inputs=++|
  Out1 : Outport
  wires:
  Step24/1 -> Sum96/2
  Step20/1 -> Sum96/1
  Sum96/1 -> Out1/1

== system pid_adrc_duibi/同7 ==
  Step20 : Step  Time=3  After=r  SampleTime=0
  Step24 : Step  Time=4  After=-r  SampleTime=0
  Sum96 : Sum  Inputs=++|
  Out1 : Outport
  wires:
  Step24/1 -> Sum96/2
  Step20/1 -> Sum96/1
  Sum96/1 -> Out1/1

== system pid_adrc_duibi/相反 ==
  Step22 : Step  Time=3  After=-r  SampleTime=0
  Step23 : Step  Time=4  After=r  SampleTime=0
  Sum110 : Sum  Inputs=++|
  Out1 : Outport
  wires:
  Step22/1 -> Sum110/1
  Step23/1 -> Sum110/2
  Sum110/1 -> Out1/1

== system pid_adrc_duibi/相反1 ==
  Step22 : Step  Time=3  After=-r  SampleTime=0
  Step23 : Step  Time=4  After=r  SampleTime=0
  Sum110 : Sum  Inputs=++|
  Out1 : Outport
  wires:
  Step22/1 -> Sum110/1
  Step23/1 -> Sum110/2
  Sum110/1 -> Out1/1

== system pid_adrc_duibi/相反2 ==
  Step22 : Step  Time=3  After=-r  SampleTime=0
  Step23 : Step  Time=4  After=r  SampleTime=0
  Sum110 : Sum  Inputs=++|
  Out1 : Outport
  wires:
  Step22/1 -> Sum110/1
  Step23/1 -> Sum110/2
  Sum110/1 -> Out1/1

== system pid_adrc_duibi/相反3 ==
  Step22 : Step  Time=3  After=-r  SampleTime=0
  Step23 : Step  Time=4  After=r  SampleTime=0
  Sum110 : Sum  Inputs=++|
  Out1 : Outport
  wires:
  Step22/1 -> Sum110/1
  Step23/1 -> Sum110/2
  Sum110/1 -> Out1/1

== system pid_adrc_duibi/相反4 ==
  Step22 : Step  Time=3  After=-r  SampleTime=0
  Step23 : Step  Time=4  After=r  SampleTime=0
  Sum110 : Sum  Inputs=++|
  Out1 : Outport
  wires:
  Step22/1 -> Sum110/1
  Step23/1 -> Sum110/2
  Sum110/1 -> Out1/1

== system pid_adrc_duibi/相反5 ==
  Step22 : Step  Time=3  After=-r  SampleTime=0
  Step23 : Step  Time=4  After=r  SampleTime=0
  Sum110 : Sum  Inputs=++|
  Out1 : Outport
  wires:
  Step22/1 -> Sum110/1
  Step23/1 -> Sum110/2
  Sum110/1 -> Out1/1

== system pid_adrc_duibi/相反6 ==
  Step22 : Step  Time=3  After=-r  SampleTime=0
  Step23 : Step  Time=4  After=r  SampleTime=0
  Sum110 : Sum  Inputs=++|
  Out1 : Outport
  wires:
  Step22/1 -> Sum110/1
  Step23/1 -> Sum110/2
  Sum110/1 -> Out1/1

== system pid_adrc_duibi/相反7 ==
  Step22 : Step  Time=3  After=-r  SampleTime=0
  Step23 : Step  Time=4  After=r  SampleTime=0
  Sum110 : Sum  Inputs=++|
  Out1 : Outport
  wires:
  Step22/1 -> Sum110/1
  Step23/1 -> Sum110/2
  Sum110/1 -> Out1/1

== matlab function pid_adrc_duibi/滑动摩擦模型1 ==
  data: f1 output; f2 output; y input
function [f1, f2]= fcn(y)
m1=18.526;       %横梁质量kg
m2=3.923;      %负载质量kg
l=0.97;    %0.97m
u=0.005;    %库伦摩擦系数u=0.005
g=9.8;

f1=u*(m1*g/2+(1/2-y/l)*m2*g);   %X1摩檫力
f2=u*(m1*g/2+(1/2+y/l)*m2*g);   %X2摩檫力

== matlab function pid_adrc_duibi/前馈补偿3 ==
  data: y input; meq1 output; meq2 output
function [meq1,meq2]= fcn(y)
m1=18.526;       %横梁质量kg
m2=3.923;      %负载质量kg
l=0.97;    %0.97m

I1=m1*l^2/12;

meq1 = (m1+m2)/2+2*(I1+m2*y^2)/l^2;
meq2 = (m1+m2)/2+2*(I1+m2*y^2)/(l-y)^2;

== matlab function pid_adrc_duibi/滑动摩擦模型5 ==
  data: f1 output; f2 output; y input
function [f1, f2]= fcn(y)
m1=18.526;       %横梁质量kg
m2=3.923;      %负载质量kg
l=0.97;    %0.97m
u=0.005;    %库伦摩擦系数u=0.005
g=9.8;

f1=u*(m1*g/2+(1/2-y/l)*m2*g);   %X1摩檫力
f2=u*(m1*g/2+(1/2+y/l)*m2*g);   %X2摩檫力

== matlab function pid_adrc_duibi/滑动摩擦模型6 ==
  data: f1 output; f2 output; y input
function [f1, f2]= fcn(y)
m1=18.526;       %横梁质量kg
m2=3.923;      %负载质量kg
l=0.97;    %0.97m
u=0.005;    %库伦摩擦系数u=0.005
g=9.8;

f1=u*(m1*g/2+(1/2-y/l)*m2*g);   %X1摩檫力
f2=u*(m1*g/2+(1/2+y/l)*m2*g);   %X2摩檫力

== matlab function pid_adrc_duibi/滑动摩擦模型7 ==
  data: f1 output; f2 output; y input
function [f1, f2]= fcn(y)
m1=18.526;       %横梁质量kg
m2=3.923;      %负载质量kg
l=0.97;    %0.97m
u=0.005;    %库伦摩擦系数u=0.005
g=9.8;

f1=u*(m1*g/2+(1/2-y/l)*m2*g);   %X1摩檫力
f2=u*(m1*g/2+(1/2+y/l)*m2*g);   %X2摩檫力

== matlab function pid_adrc_duibi/滑动摩擦模型8 ==
  data: f1 output; f2 output; y input
function [f1, f2]= fcn(y)
m1=18.526;       %横梁质量kg
m2=3.923;      %负载质量kg
l=0.97;    %0.97m
u=0.005;    %库伦摩擦系数u=0.005
g=9.8;

f1=u*(m1*g/2+(1/2-y/l)*m2*g);   %X1摩檫力
f2=u*(m1*g/2+(1/2+y/l)*m2*g);   %X2摩檫力

== matlab function pid_adrc_duibi/龙门平台5 ==
  data: out1 output; u1 input; y input; out2 output; u2 input
function [out1, out2]= fcn(u1, y, u2)
m1=18.526;       %横梁质量kg
m2=3.923;      %负载质量kg
l=0.97;    %0.97m


I1=m1*l^2/12;   %转动惯量



%动力学方程
%U= m2^2*y^2+2*m1*m2*y^2+I1*(m1+m2);
Q11=(2*m2*y^2+m2*l*y+I1+l^2*(m1+m2)/4);       
Q12=(2*m2*y^2++I1-l^2*(m1+m2)/4);
Q21=(2*m2*y^2++I1-l^2*(m1+m2)/4);
Q22=(2*m2*y^2-m2*l*y+I1+l^2*(m1+m2)/4);


out1=u1*Q11+u2*Q21;
out2=u1*Q12+u2*Q22;

== matlab function pid_adrc_duibi/龙门平台6 ==
  data: out1 output; u1 input; y input; out2 output; u2 input
function [out1, out2]= fcn(u1, y, u2)
m1=18.526;       %横梁质量kg
m2=3.923;      %负载质量kg
l=0.97;    %0.97m


I1=m1*l^2/12;   %转动惯量



%动力学方程
U= m2^2*y^2+2*m1*m2*y^2+I1*(m1+m2);
Q11=(2*m2*y^2+m2*l*y+I1+l^2*(m1+m2)/4);       
Q12=(2*m2*y^2++I1-l^2*(m1+m2)/4);
Q21=(2*m2*y^2++I1-l^2*(m1+m2)/4);
Q22=(2*m2*y^2-m2*l*y+I1+l^2*(m1+m2)/4);


out1=u1*Q11+u2*Q21;
out2=u1*Q12+u2*Q22;

== matlab function pid_adrc_duibi/龙门平台7 ==
  data: out1 output; u1 input; y input; out2 output; u2 input
function [out1, out2]= fcn(u1, y, u2)
m1=18.526;       %横梁质量kg
m2=3.923;      %负载质量kg
l=0.97;    %0.97m


I1=m1*l^2/12;   %转动惯量



%动力学方程
U= m2^2*y^2+2*m1*m2*y^2+I1*(m1+m2);
Q11=(2*m2*y^2+m2*l*y+I1+l^2*(m1+m2)/4);       
Q12=(2*m2*y^2++I1-l^2*(m1+m2)/4);
Q21=(2*m2*y^2++I1-l^2*(m1+m2)/4);
Q22=(2*m2*y^2-m2*l*y+I1+l^2*(m1+m2)/4);


out1=u1*Q11+u2*Q21;
out2=u1*Q12+u2*Q22;

== matlab function pid_adrc_duibi/龙门平台8 ==
  data: out1 output; u1 input; y input; out2 output; u2 input
function [out1, out2]= fcn(u1, y, u2)
m1=18.526;       %横梁质量kg
m2=3.923;      %负载质量kg
l=0.97;    %0.97m


I1=m1*l^2/12;   %转动惯量



%动力学方程
U= m2^2*y^2+2*m1*m2*y^2+I1*(m1+m2);
Q11=(2*m2*y^2+m2*l*y+I1+l^2*(m1+m2)/4)/U;       
Q12=(2*m2*y^2++I1-l^2*(m1+m2)/4)/U;
Q21=(2*m2*y^2++I1-l^2*(m1+m2)/4)/U;
Q22=(2*m2*y^2-m2*l*y+I1+l^2*(m1+m2)/4)/U;


out1=u1*Q11+u2*Q21;
out2=u1*Q12+u2*Q22;

== matlab function pid_adrc_duibi/滑动摩擦模型4 ==
  data: f1 output; f2 output; y input
function [f1, f2]= fcn(y)
m1=18.526;       %横梁质量kg
m2=3.923;      %负载质量kg
l=0.97;    %0.97m
u=0.005;    %库伦摩擦系数u=0.005
g=9.8;

f1=u*(m1*g/2+(1/2-y/l)*m2*g);   %X1摩檫力
f2=u*(m1*g/2+(1/2+y/l)*m2*g);   %X2摩檫力

== matlab function pid_adrc_duibi/前馈补偿 ==
  data: y input; meq1 output; meq2 output
function [meq1,meq2]= fcn(y)
m1=18.526;       %横梁质量kg
m2=3.923;      %负载质量kg
l=0.97;    %0.97m

I1=m1*l^2/12;

meq1 = (m1+m2)/2+2*(I1+m2*y^2)/l^2;
meq2 = (m1+m2)/2+2*(I1+m2*y^2)/(l-y)^2;

== matlab function pid_adrc_duibi/前馈补偿2 ==
  data: y input; meq1 output; meq2 output
function [meq1,meq2]= fcn(y)
m1=18.526;       %横梁质量kg
m2=3.923;      %负载质量kg
l=0.97;    %0.97m

I1=m1*l^2/12;

meq1 = (m1+m2)/2+2*(I1+m2*y^2)/l^2;
meq2 = (m1+m2)/2+2*(I1+m2*y^2)/(l-y)^2;

== matlab function pid_adrc_duibi/滑动摩擦模型2 ==
  data: f1 output; f2 output; y input
function [f1, f2]= fcn(y)
m1=18.526;       %横梁质量kg
m2=3.923;      %负载质量kg
l=0.97;    %0.97m
u=0.005;    %库伦摩擦系数u=0.005
g=9.8;

f1=u*(m1*g/2+(1/2-y/l)*m2*g);   %X1摩檫力
f2=u*(m1*g/2+(1/2+y/l)*m2*g);   %X2摩檫力

== matlab function pid_adrc_duibi/前馈补偿1 ==
  data: y input; meq1 output; meq2 output
function [meq1,meq2]= fcn(y)
m1=18.526;       %横梁质量kg
m2=3.923;      %负载质量kg
l=0.97;    %0.97m

I1=m1*l^2/12;

meq1 = (m1+m2)/2+2*(I1+m2*y^2)/l^2;
meq2 = (m1+m2)/2+2*(I1+m2*y^2)/(l-y)^2;

== matlab function pid_adrc_duibi/龙门平台1 ==
  data: out1 output; u1 input; y input; out2 output; u2 input
function [out1, out2]= fcn(u1, y, u2)
m1=18.526;       %横梁质量kg
m2=3.923;      %负载质量kg
l=0.97;    %0.97m


I1=m1*l^2/12;   %转动惯量



%动力学方程
%U= m2^2*y^2+2*m1*m2*y^2+I1*(m1+m2);
Q11=(2*m2*y^2+m2*l*y+I1+l^2*(m1+m2)/4);       
Q12=(2*m2*y^2++I1-l^2*(m1+m2)/4);
Q21=(2*m2*y^2++I1-l^2*(m1+m2)/4);
Q22=(2*m2*y^2-m2*l*y+I1+l^2*(m1+m2)/4);


out1=u1*Q11+u2*Q21;
out2=u1*Q12+u2*Q22;

== matlab function pid_adrc_duibi/滑动摩擦模型3 ==
  data: f1 output; f2 output; y input
function [f1, f2]= fcn(y)
m1=18.526;       %横梁质量kg
m2=3.923;      %负载质量kg
l=0.97;    %0.97m
u=0.005;    %库伦摩擦系数u=0.005
g=9.8;

f1=u*(m1*g/2+(1/2-y/l)*m2*g);   %X1摩檫力
f2=u*(m1*g/2+(1/2+y/l)*m2*g);   %X2摩檫力

== matlab function pid_adrc_duibi/龙门平台3 ==
  data: out1 output; u1 input; y input; out2 output; u2 input
function [out1, out2]= fcn(u1, y, u2)
m1=18.526;       %横梁质量kg
m2=3.923;      %负载质量kg
l=0.97;    %0.97m


I1=m1*l^2/12;   %转动惯量



%动力学方程
U= m2^2*y^2+2*m1*m2*y^2+I1*(m1+m2);
Q11=(2*m2*y^2+m2*l*y+I1+l^2*(m1+m2)/4);       
Q12=(2*m2*y^2++I1-l^2*(m1+m2)/4);
Q21=(2*m2*y^2++I1-l^2*(m1+m2)/4);
Q22=(2*m2*y^2-m2*l*y+I1+l^2*(m1+m2)/4);


out1=u1*Q11+u2*Q21;
out2=u1*Q12+u2*Q22;

== matlab function pid_adrc_duibi/龙门平台4 ==
  data: out1 output; u1 input; y input; out2 output; u2 input
function [out1, out2]= fcn(u1, y, u2)
m1=18.526;       %横梁质量kg
m2=3.923;      %负载质量kg
l=0.97;    %0.97m


I1=m1*l^2/12;   %转动惯量



%动力学方程
U= m2^2*y^2+2*m1*m2*y^2+I1*(m1+m2);
Q11=(2*m2*y^2+m2*l*y+I1+l^2*(m1+m2)/4)/U;       
Q12=(2*m2*y^2++I1-l^2*(m1+m2)/4)/U;
Q21=(2*m2*y^2++I1-l^2*(m1+m2)/4)/U;
Q22=(2*m2*y^2-m2*l*y+I1+l^2*(m1+m2)/4)/U;


out1=u1*Q11+u2*Q21;
out2=u1*Q12+u2*Q22;

== matlab function pid_adrc_duibi/龙门平台2 ==
  data: out1 output; u1 input; y input; out2 output; u2 input
function [out1, out2]= fcn(u1, y, u2)
m1=18.526;       %横梁质量kg
m2=3.923;      %负载质量kg
l=0.97;    %0.97m


I1=m1*l^2/12;   %转动惯量



%动力学方程
U= m2^2*y^2+2*m1*m2*y^2+I1*(m1+m2);
Q11=(2*m2*y^2+m2*l*y+I1+l^2*(m1+m2)/4);       
Q12=(2*m2*y^2++I1-l^2*(m1+m2)/4);
Q21=(2*m2*y^2++I1-l^2*(m1+m2)/4);
Q22=(2*m2*y^2-m2*l*y+I1+l^2*(m1+m2)/4);


out1=u1*Q11+u2*Q21;
out2=u1*Q12+u2*Q22;
